simulink model "Distribution_longestqueue"  (Simulink 7.9)
settings: Solver=VariableStepDiscrete  StartTime=0.0  StopTime=500  RelTol=1e-3
libraries: simeventslib x13
(part 2 of 2)

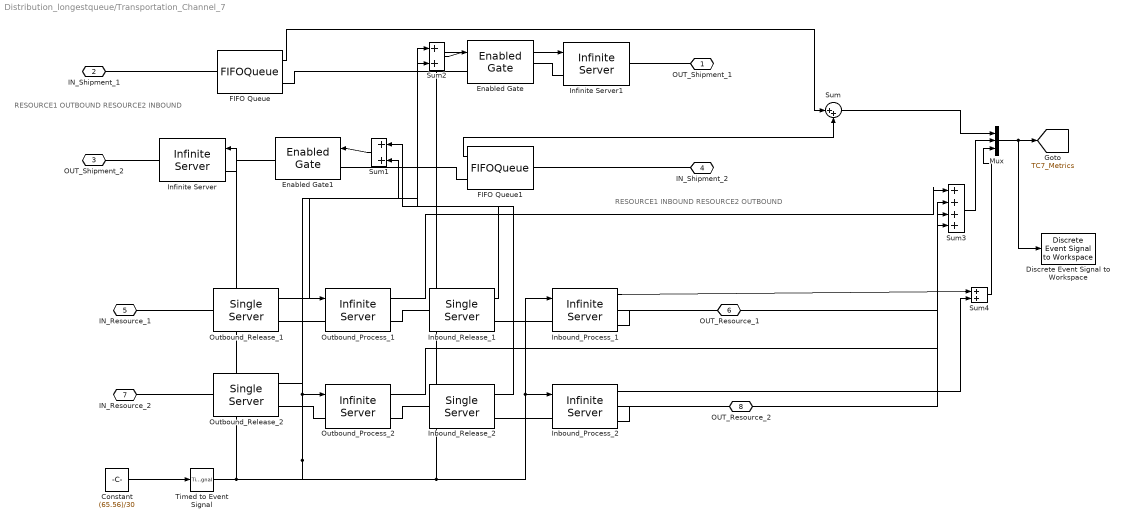
== system Distribution_longestqueue/Transportation_Channel_7 ==
  note: RESOURCE1 INBOUND
      | RESOURCE2 OUTBOUND
  note: RESOURCE1 OUTBOUND
      | RESOURCE2 INBOUND
  Constant : Constant  Value=(65.56)/30
  Discrete Event Signal to Workspace : simeventslib/SimEvents Sinks/Discrete Event Signal to Workspace  VariableName=TC7_Status  SaveFormat=Structure With Time  isMonitorOnly=off  isRecordIC=off
  Enabled Gate : EnabledGate
  Enabled Gate1 : EnabledGate
  FIFO Queue : FIFOQueue  Capacity=inf  StatNumberInBlock=on
      settings: OutputPortMap=o1
  FIFO Queue1 : FIFOQueue  Capacity=inf  StatNumberInBlock=on
      settings: OutputPortMap=o1
  Inbound_Process_1 : InfiniteServer  ServiceTimeFrom=Signal port t  ServiceTime=(76.7)/30  StatNumberDeparted=on  StatNumberInBlock=on
      settings: OutputPortMap=o0,o1
  Inbound_Process_2 : InfiniteServer  ServiceTimeFrom=Signal port t  ServiceTime=(76.7)/30  StatNumberDeparted=on  StatNumberInBlock=on
      settings: OutputPortMap=o0,o1
  Inbound_Release_1 : SingleServer  ServiceTime=0  StatNumberInBlock=on
      settings: OutputPortMap=o1
  Inbound_Release_2 : SingleServer  ServiceTime=0  StatNumberInBlock=on
      settings: OutputPortMap=o1
  Infinite Server : InfiniteServer  ServiceTimeFrom=Signal port t  ServiceTime=(76.7)/30
  Infinite Server1 : InfiniteServer  ServiceTimeFrom=Signal port t  ServiceTime=(76.7)/30
  Mux : Mux  Inputs=3
  Outbound_Process_1 : InfiniteServer  ServiceTimeFrom=Signal port t  ServiceTime=(76.7)/30  StatNumberInBlock=on
      settings: OutputPortMap=o1
  Outbound_Process_2 : InfiniteServer  ServiceTimeFrom=Signal port t  ServiceTime=(76.7)/30  StatNumberInBlock=on
      settings: OutputPortMap=o1
  Outbound_Release_1 : SingleServer  ServiceTime=0  StatNumberInBlock=on
      settings: OutputPortMap=o1
  Outbound_Release_2 : SingleServer  ServiceTime=0  StatNumberInBlock=on
      settings: OutputPortMap=o1
  Sum{,1..2,4} (4 alike) : Sum  Inputs=|++
  Sum3 : Sum  Inputs=|++++
  Timed to Event Signal : TimedToEventSignal
  OUT_Shipment_1 : PMIOPort  Port=1  Side=Right
  IN_Shipment_1 : PMIOPort  Port=2  Side=Right
  OUT_Shipment_2 : PMIOPort  Port=3  Side=Left
  IN_Shipment_2 : PMIOPort  Port=4  Side=Left
  IN_Resource_1 : PMIOPort  Port=5  Side=Right
  OUT_Resource_1 : PMIOPort  Port=6  Side=Right
  IN_Resource_2 : PMIOPort  Port=7  Side=Left
  OUT_Resource_2 : PMIOPort  Port=8  Side=Left
  tag scope: TC7_Metrics=global
  wires:
  FIFO Queue1/1 -> Sum/2
  FIFO Queue/1 -> Sum/1
  Sum/1 -> Mux/1
  Constant/1 -> Timed to Event Signal/1
  Timed to Event Signal/1 -> Outbound_Process_1/1, Outbound_Process_2/1, Inbound_Process_1/1, Inbound_Process_2/1, Infinite Server1/1, Infinite Server/1
  Sum1/1 -> Enabled Gate1/1
  Outbound_Release_2/1 -> Sum1/2
  Inbound_Release_1/1 -> Sum1/1
  Sum2/1 -> Enabled Gate/1
  Outbound_Release_1/1 -> Sum2/1
  Inbound_Release_2/1 -> Sum2/2
  Mux/1 -> [TC7_Metrics], Discrete Event Signal to Workspace/1
  Sum3/1 -> Mux/2
  Outbound_Process_1/1 -> Sum3/1
  Inbound_Process_1/2 -> Sum3/2
  Outbound_Process_2/1 -> Sum3/3
  Inbound_Process_2/2 -> Sum3/4
  Inbound_Process_2/1 -> Sum4/2
  Inbound_Process_1/1 -> Sum4/1
  Sum4/1 -> Mux/3
  connections:
  FIFO Queue/RConn1 -- Enabled Gate/LConn1
  Enabled Gate1/LConn1 -- FIFO Queue1/RConn1
  IN_Shipment_1/RConn1 -- FIFO Queue/LConn1
  IN_Shipment_2/RConn1 -- FIFO Queue1/LConn1
  IN_Resource_1/RConn1 -- Outbound_Release_1/LConn1
  OUT_Shipment_2/RConn1 -- Infinite Server/RConn1
  Infinite Server/LConn1 -- Enabled Gate1/RConn1
  Enabled Gate/RConn1 -- Infinite Server1/LConn1
  Infinite Server1/RConn1 -- OUT_Shipment_1/RConn1
  IN_Resource_2/RConn1 -- Outbound_Release_2/LConn1
  Outbound_Release_2/RConn1 -- Outbound_Process_2/LConn1
  Outbound_Process_2/RConn1 -- Inbound_Release_2/LConn1
  Inbound_Release_2/RConn1 -- Inbound_Process_2/LConn1
  Inbound_Process_2/RConn1 -- OUT_Resource_2/RConn1
  Outbound_Release_1/RConn1 -- Outbound_Process_1/LConn1
  Inbound_Release_1/RConn1 -- Inbound_Process_1/LConn1
  Outbound_Process_1/RConn1 -- Inbound_Release_1/LConn1
  Inbound_Process_1/RConn1 -- OUT_Resource_1/RConn1

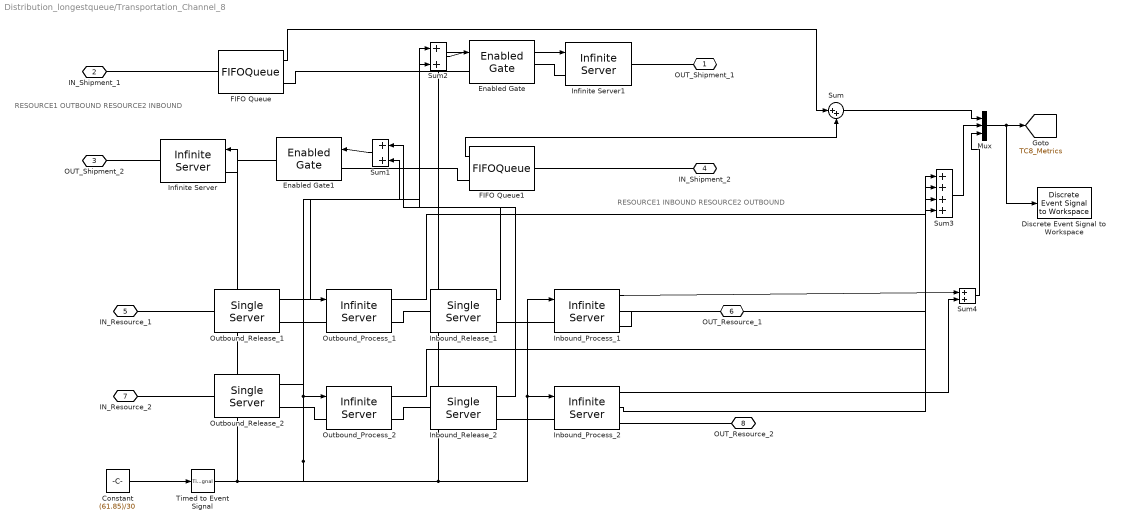
== system Distribution_longestqueue/Transportation_Channel_8 ==
  note: RESOURCE1 INBOUND
      | RESOURCE2 OUTBOUND
  note: RESOURCE1 OUTBOUND
      | RESOURCE2 INBOUND
  Constant : Constant  Value=(61.85)/30
  Discrete Event Signal to Workspace : simeventslib/SimEvents Sinks/Discrete Event Signal to Workspace  VariableName=TC8_Status  SaveFormat=Structure With Time  isMonitorOnly=off  isRecordIC=off
  Enabled Gate : EnabledGate
  Enabled Gate1 : EnabledGate
  FIFO Queue : FIFOQueue  Capacity=inf  StatNumberInBlock=on
      settings: OutputPortMap=o1
  FIFO Queue1 : FIFOQueue  Capacity=inf  StatNumberInBlock=on
      settings: OutputPortMap=o1
  Inbound_Process_1 : InfiniteServer  ServiceTimeFrom=Signal port t  ServiceTime=(76.7)/30  StatNumberDeparted=on  StatNumberInBlock=on
      settings: OutputPortMap=o0,o1
  Inbound_Process_2 : InfiniteServer  ServiceTimeFrom=Signal port t  ServiceTime=(76.7)/30  StatNumberDeparted=on  StatNumberInBlock=on
      settings: OutputPortMap=o0,o1
  Inbound_Release_1 : SingleServer  ServiceTime=0  StatNumberInBlock=on
      settings: OutputPortMap=o1
  Inbound_Release_2 : SingleServer  ServiceTime=0  StatNumberInBlock=on
      settings: OutputPortMap=o1
  Infinite Server : InfiniteServer  ServiceTimeFrom=Signal port t  ServiceTime=(76.7)/30
  Infinite Server1 : InfiniteServer  ServiceTimeFrom=Signal port t  ServiceTime=(76.7)/30
  Mux : Mux  Inputs=3
  Outbound_Process_1 : InfiniteServer  ServiceTimeFrom=Signal port t  ServiceTime=(76.7)/30  StatNumberInBlock=on
      settings: OutputPortMap=o1
  Outbound_Process_2 : InfiniteServer  ServiceTimeFrom=Signal port t  ServiceTime=(76.7)/30  StatNumberInBlock=on
      settings: OutputPortMap=o1
  Outbound_Release_1 : SingleServer  ServiceTime=0  StatNumberInBlock=on
      settings: OutputPortMap=o1
  Outbound_Release_2 : SingleServer  ServiceTime=0  StatNumberInBlock=on
      settings: OutputPortMap=o1
  Sum{,1..2,4} (4 alike) : Sum  Inputs=|++
  Sum3 : Sum  Inputs=|++++
  Timed to Event Signal : TimedToEventSignal
  OUT_Shipment_1 : PMIOPort  Port=1  Side=Right
  IN_Shipment_1 : PMIOPort  Port=2  Side=Right
  OUT_Shipment_2 : PMIOPort  Port=3  Side=Left
  IN_Shipment_2 : PMIOPort  Port=4  Side=Left
  IN_Resource_1 : PMIOPort  Port=5  Side=Right
  OUT_Resource_1 : PMIOPort  Port=6  Side=Right
  IN_Resource_2 : PMIOPort  Port=7  Side=Left
  OUT_Resource_2 : PMIOPort  Port=8  Side=Left
  tag scope: TC8_Metrics=global
  wires:
  FIFO Queue1/1 -> Sum/2
  FIFO Queue/1 -> Sum/1
  Sum/1 -> Mux/1
  Constant/1 -> Timed to Event Signal/1
  Timed to Event Signal/1 -> Outbound_Process_1/1, Outbound_Process_2/1, Inbound_Process_1/1, Inbound_Process_2/1, Infinite Server1/1, Infinite Server/1
  Sum1/1 -> Enabled Gate1/1
  Outbound_Release_2/1 -> Sum1/2
  Inbound_Release_1/1 -> Sum1/1
  Sum2/1 -> Enabled Gate/1
  Outbound_Release_1/1 -> Sum2/1
  Inbound_Release_2/1 -> Sum2/2
  Mux/1 -> [TC8_Metrics], Discrete Event Signal to Workspace/1
  Sum3/1 -> Mux/2
  Outbound_Process_1/1 -> Sum3/1
  Inbound_Process_1/2 -> Sum3/2
  Outbound_Process_2/1 -> Sum3/3
  Inbound_Process_2/2 -> Sum3/4
  Sum4/1 -> Mux/3
  Inbound_Process_1/1 -> Sum4/1
  Inbound_Process_2/1 -> Sum4/2
  connections:
  FIFO Queue/RConn1 -- Enabled Gate/LConn1
  Enabled Gate1/LConn1 -- FIFO Queue1/RConn1
  IN_Shipment_1/RConn1 -- FIFO Queue/LConn1
  IN_Shipment_2/RConn1 -- FIFO Queue1/LConn1
  IN_Resource_1/RConn1 -- Outbound_Release_1/LConn1
  OUT_Shipment_2/RConn1 -- Infinite Server/RConn1
  Infinite Server/LConn1 -- Enabled Gate1/RConn1
  Enabled Gate/RConn1 -- Infinite Server1/LConn1
  Infinite Server1/RConn1 -- OUT_Shipment_1/RConn1
  IN_Resource_2/RConn1 -- Outbound_Release_2/LConn1
  Outbound_Release_2/RConn1 -- Outbound_Process_2/LConn1
  Outbound_Process_2/RConn1 -- Inbound_Release_2/LConn1
  Inbound_Release_2/RConn1 -- Inbound_Process_2/LConn1
  Inbound_Process_2/RConn1 -- OUT_Resource_2/RConn1
  Outbound_Release_1/RConn1 -- Outbound_Process_1/LConn1
  Inbound_Release_1/RConn1 -- Inbound_Process_1/LConn1
  Outbound_Process_1/RConn1 -- Inbound_Release_1/LConn1
  Inbound_Process_1/RConn1 -- OUT_Resource_1/RConn1

== system Distribution_longestqueue/Depot_10/Resource_Pool ==
  Event-Based Entity Generator : EventBasedEntityGenerator  GenerateEntitiesUpon=Function call from port fcn
  FIFO Queue : FIFOQueue  Capacity=8
  Path Combiner : PathCombiner  NumberInputPorts=2
  Time-Based Function-Call Generator : TimeBasedFunctionCallGenerator  EventGenerationMode=Only at simulation start  NumberOfEventsPerPeriod=Quantity
  Acquire : PMIOPort  Port=1  Side=Left
  Return : PMIOPort  Port=2  Side=Right
  wires:
  Time-Based Function-Call Generator/1 -> Event-Based Entity Generator/1
  connections:
  Event-Based Entity Generator/RConn1 -- Path Combiner/LConn1
  Path Combiner/RConn1 -- FIFO Queue/LConn1
  Return/RConn1 -- Path Combiner/LConn2
  Acquire/RConn1 -- FIFO Queue/RConn1

== system Distribution_longestqueue/Depot_6/Resource_Pool ==
  Event-Based Entity Generator : EventBasedEntityGenerator  GenerateEntitiesUpon=Function call from port fcn
  FIFO Queue : FIFOQueue  Capacity=8
  Path Combiner : PathCombiner  NumberInputPorts=2
  Time-Based Function-Call Generator : TimeBasedFunctionCallGenerator  EventGenerationMode=Only at simulation start  NumberOfEventsPerPeriod=Quantity
  Acquire : PMIOPort  Port=1  Side=Left
  Return : PMIOPort  Port=2  Side=Right
  wires:
  Time-Based Function-Call Generator/1 -> Event-Based Entity Generator/1
  connections:
  Event-Based Entity Generator/RConn1 -- Path Combiner/LConn1
  Path Combiner/RConn1 -- FIFO Queue/LConn1
  Return/RConn1 -- Path Combiner/LConn2
  Acquire/RConn1 -- FIFO Queue/RConn1

== system Distribution_longestqueue/Depot_9/Resource_Pool ==
  Event-Based Entity Generator : EventBasedEntityGenerator  GenerateEntitiesUpon=Function call from port fcn
  FIFO Queue : FIFOQueue  Capacity=8
  Path Combiner : PathCombiner  NumberInputPorts=2
  Time-Based Function-Call Generator : TimeBasedFunctionCallGenerator  EventGenerationMode=Only at simulation start  NumberOfEventsPerPeriod=Quantity
  Acquire : PMIOPort  Port=1  Side=Left
  Return : PMIOPort  Port=2  Side=Right
  wires:
  Time-Based Function-Call Generator/1 -> Event-Based Entity Generator/1
  connections:
  Event-Based Entity Generator/RConn1 -- Path Combiner/LConn1
  Path Combiner/RConn1 -- FIFO Queue/LConn1
  Return/RConn1 -- Path Combiner/LConn2
  Acquire/RConn1 -- FIFO Queue/RConn1

== matlab function Depot_10/MATLAB Function ==
  data: route input double; next output double; current input double
function next = routing(route, current)
%#codegen
next = 1;
for i = 1:length(route)
   if route(i) == current
       next = route(i+1);
   end
end

== matlab function Depot_6/MATLAB Function ==
  data: route input double; next output double; current input double
function next = routing(route, current)
%#codegen

next= 1;
for i = 1:length(route)
   if route(i) == current
       next = route(i+1);
   end
end

== matlab function Depot_9/MATLAB Function ==
  data: route input double; next output double; current input double
function next = routing(route, current)
%#codegen

next = 1;
for i = 1:length(route)
   if route(i) == current
       next = route(i+1);
   end
end

== matlab function Depot_10/Control: Resource Allocation ==
  data: IN_1 input double; OUT_1 output double; IN_2 input double; IN_3 input double; IN_4 input double
function OUT_1 = resource_alloc(IN_1, IN_2, IN_3, IN_4)
%#codegen

OUT_1 = 1;

Status = [IN_1'; IN_2'; IN_3'; IN_4'];

y = min(Status(:,2));
x = max(Status(Status(:,2)==y));

for i = 1:length(Status(:,1))
   if Status(i,1)== x && Status(i,2) == y
       OUT_1 = i;
       break;
   end
end

== matlab function Depot_9/MATLAB Function1 ==
  data: IN_1 input double; OUT_1 output double; IN_2 input double; IN_3 input double; IN_4 input double
function OUT_1 = resource_alloc(IN_1, IN_2, IN_3, IN_4)
%#codegen

OUT_1 = 1;

Status = [IN_1'; IN_2'; IN_3'; IN_4'];

y = min(Status(:,2));
x = max(Status(Status(:,2)==y));

for i = 1:length(Status(:,1))
   if Status(i,1)== x && Status(i,2) == y
       OUT_1 = i;
       break;
   end
end

== matlab function Depot_6/MATLAB Function1 ==
  data: IN_1 input double; OUT_1 output double; IN_2 input double; IN_3 input double
function OUT_1 = resource_alloc(IN_1, IN_2, IN_3)
%#codegen

OUT_1 = 1;

Status = [IN_1'; IN_2'; IN_3'];

y = min(Status(:,2));
x = max(Status(Status(:,2)==y));

for i = 1:length(Status(:,1))
   if Status(i,1)== x && Status(i,2) == y
       OUT_1 = i;
       break;
   end
end
